simulink model "RefModel_magCalib_memoryGood"  (R2020b)
settings: Solver=FixedStepDiscrete  StartTime=0.0  StopTime=inf  FixedStep=Ts  RelTol=1e-3
model workspace (MAT data in the model file):
  Tf = 231.9
  Ts = 0.012
  xSim1.time = [0 0.012 0.024 0.036 0.048 0.06 0.072 0.084 0.096 0.108 0.12 0.132 ... (19326 elements, 1x19326)]
  xSim1.signals.values = [0.0833129882812 0.0833129882812 0.078857421875 0.0801391601562 0.0801391601562 0.07763671875 0.07470703125 0.07470703125 0.0751342773438 0.07763671875 0.07763671875 0.0755615234375 ... (57978 elements, 19326x3)]
  xSim1.signals.dimensions = 3
  xSim2.time = [0 0.012 0.024 0.036 0.048 0.06 0.072 0.084 0.096 0.108 0.12 0.132 ... (19326 elements, 1x19326)]
  xSim2.signals.values = [0.167907714844 0.167907714844 0.176208496094 0.172912597656 0.172912597656 0.17431640625 0.178894042969 0.178894042969 0.174743652344 0.173278808594 0.173278808594 0.176208496094 ... (57978 elements, 19326x3)]
  xSim2.signals.dimensions = 3
settings Model: PauseTimes=66  PacingRate=0.011000  Creator=sl  LastModifiedBy=sl
settings OptimizationCC: DefaultParameterBehavior=Inlined  EnhancedBackFolding=on  PassReuseOutputArgsAs=Individual arguments  ZeroExternalMemoryAtStartup=off  ZeroInternalMemoryAtStartup=off  MaxStackSize=64  OptimizeBlockOrder=speed  DifferentSizesBufferReuse=on  OptimizationCustomize=off  EfficientTunableParamExpr=on
settings DebuggingCC: ParameterTunabilityLossMsg=error
settings HardwareCC: ProdBitPerPointer=32  ProdBitPerSizeT=32  ProdBitPerPtrDiffT=32  ProdLargestAtomicInteger=Long  ProdLargestAtomicFloat=Double  ProdWordSize=32  ProdHWDeviceType=ARM Compatible->ARM Cortex
settings SFSimCC: MATLABDynamicMemAlloc=off
settings RTWCC: Description=Embedded Coder  SystemTargetFile=ert.tlc  GenCodeOnly=on  PackageGeneratedCodeAndArtifacts=on  TemplateMakefile=ert_default_tmf  GenerateReport=on  IncludeHyperlinkInReport=on  LaunchReport=on  GenerateTraceInfo=on  GenerateTraceReport=on  GenerateTraceReportSl=on  GenerateTraceReportSf=on  GenerateTraceReportEml=on
settings CodeAppCC: ForceParamTrailComments=on  IgnoreCustomStorageClasses=off  OperatorAnnotations=on  SimulinkDataObjDesc=on  SFDataObjDesc=on  InsertBlockDesc=on
settings ERTTargetCC: SupportVariableSizeSignals=on  ERTCustomFileTemplate=example_file_process.tlc  ERTFilePackagingFormat=Compact

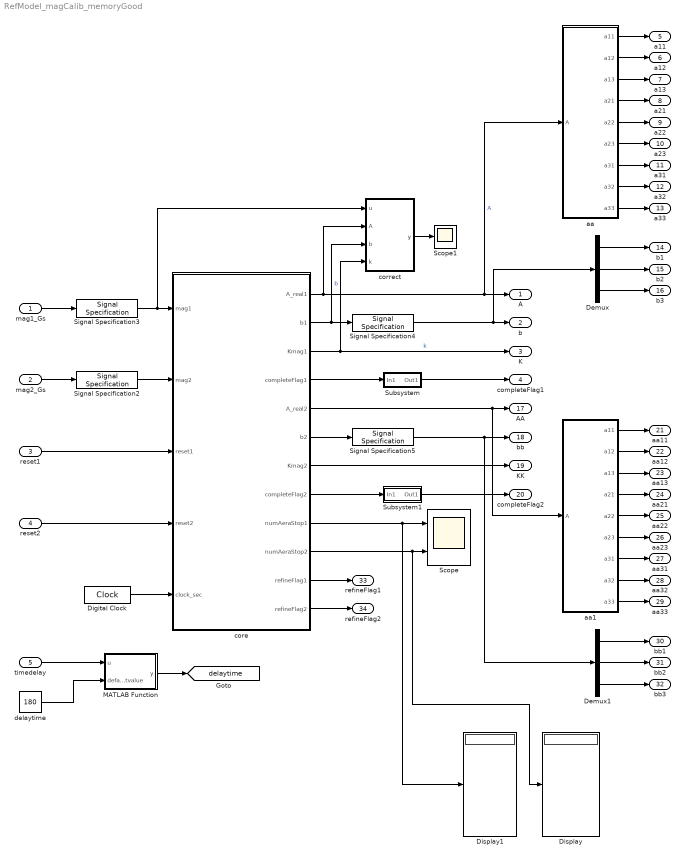
== system RefModel_magCalib_memoryGood ==
  mag1_Gs : Inport
  mag2_Gs : Inport  Port=2
  reset1 : Inport  Port=3
  reset2 : Inport  Port=4
  timedelay : Inport  Port=5
  Demux : Demux  Outputs=3
  Demux1 : Demux  Outputs=3
  Digital Clock : DigitalClock  SampleTime=-1
  Display : Display
  Display1 : Display
  MATLAB Function : MATLAB Function  TreatAsAtomicUnit=on
  Scope : Scope  NumInputPorts=2
  Scope1 : Scope
  Signal Specification{2..5} (4 alike) : SignalSpecification  OutDataTypeStr=single  Dimensions=[1,3]
  Subsystem : Subsystem
  Subsystem1 : Subsystem
  aa : MATLAB Function  TreatAsAtomicUnit=on
  aa1 : MATLAB Function  TreatAsAtomicUnit=on
  core : MATLAB Function  TreatAsAtomicUnit=on
  correct : MATLAB Function  TreatAsAtomicUnit=on
  delaytime : Constant  Value=180
  A : Outport
  b : Outport  Port=2
  K : Outport  Port=3
  completeFlag1 : Outport  Port=4
  a11 : Outport  Port=5
  a12 : Outport  Port=6
  a13 : Outport  Port=7
  a21 : Outport  Port=8
  a22 : Outport  Port=9
  a23 : Outport  Port=10
  a31 : Outport  Port=11
  a32 : Outport  Port=12
  a33 : Outport  Port=13
  b1 : Outport  Port=14
  b2 : Outport  Port=15
  b3 : Outport  Port=16
  AA : Outport  Port=17
  bb : Outport  Port=18
  KK : Outport  Port=19
  completeFlag2 : Outport  Port=20
  aa11 : Outport  Port=21
  aa12 : Outport  Port=22
  aa13 : Outport  Port=23
  aa21 : Outport  Port=24
  aa22 : Outport  Port=25
  aa23 : Outport  Port=26
  aa31 : Outport  Port=27
  aa32 : Outport  Port=28
  aa33 : Outport  Port=29
  bb1 : Outport  Port=30
  bb2 : Outport  Port=31
  bb3 : Outport  Port=32
  refineFlag1 : Outport  Port=33
  refineFlag2 : Outport  Port=34
  tag scope: delaytime=global
  wires:
  aa/2(a12) -> a12/1
  Signal Specification3/1 -> correct/1(u), core/1(mag1)
  aa/3(a13) -> a13/1
  core/1(A_real1) -> correct/2(A), aa/1(A), A/1  "A"
  aa/4(a21) -> a21/1
  core/4(completeFlag1) -> Subsystem/1(In1)
  aa/5(a22) -> a22/1
  aa/9(a33) -> a33/1
  Demux/3 -> b3/1
  Demux/1 -> b1/1
  Demux/2 -> b2/1
  aa/6(a23) -> a23/1
  aa/7(a31) -> a31/1
  aa/1(a11) -> a11/1
  core/2(b1) -> correct/3(b), Signal Specification4/1  "b"
  aa/8(a32) -> a32/1
  mag1_Gs/1 -> Signal Specification3/1
  core/3(Kmag1) -> correct/4(k), K/1  "k"
  Signal Specification2/1 -> core/2(mag2)
  mag2_Gs/1 -> Signal Specification2/1
  core/7(Kmag2) -> KK/1
  core/8(completeFlag2) -> Subsystem1/1(In1)
  aa1/3(a13) -> aa13/1
  core/6(b2) -> Signal Specification5/1
  aa1/4(a21) -> aa21/1
  aa1/9(a33) -> aa33/1
  aa1/5(a22) -> aa22/1
  aa1/8(a32) -> aa32/1
  core/5(A_real2) -> AA/1, aa1/1(A)
  aa1/7(a31) -> aa31/1
  Demux1/1 -> bb1/1
  Demux1/3 -> bb3/1
  aa1/2(a12) -> aa12/1
  Demux1/2 -> bb2/1
  aa1/1(a11) -> aa11/1
  aa1/6(a23) -> aa23/1
  reset1/1 -> core/3(reset1)
  reset2/1 -> core/4(reset2)
  Signal Specification4/1 -> Demux/1, b/1
  Signal Specification5/1 -> Demux1/1, bb/1
  core/9(numAeraStop1) -> Display1/1, Scope/1
  core/10(numAeraStop2) -> Scope/2, Display/1
  correct/1(y) -> Scope1/1
  Digital Clock/1 -> core/5(clock_sec)
  core/11(refineFlag1) -> refineFlag1/1
  core/12(refineFlag2) -> refineFlag2/1
  Subsystem/1(Out1) -> completeFlag1/1
  Subsystem1/1(Out1) -> completeFlag2/1
  timedelay/1 -> MATLAB Function/1(u)
  MATLAB Function/1(y) -> [delaytime]
  delaytime/1 -> MATLAB Function/2(defaultvalue)

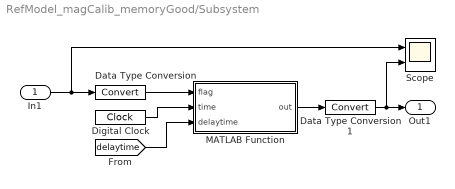
== system RefModel_magCalib_memoryGood/Subsystem ==
  In1 : Inport
  Data Type Conversion : DataTypeConversion
  Data Type Conversion1 : DataTypeConversion
  Digital Clock : DigitalClock  SampleTime=-1
  MATLAB Function : MATLAB Function  TreatAsAtomicUnit=on
  Scope : Scope  NumInputPorts=2
  Out1 : Outport
  wires:
  In1/1 -> Scope/1, Data Type Conversion/1
  MATLAB Function/1(out) -> Data Type Conversion1/1
  Digital Clock/1 -> MATLAB Function/2(time)
  Data Type Conversion/1 -> MATLAB Function/1(flag)
  Data Type Conversion1/1 -> Scope/2, Out1/1
  [delaytime] -> MATLAB Function/3(delaytime)

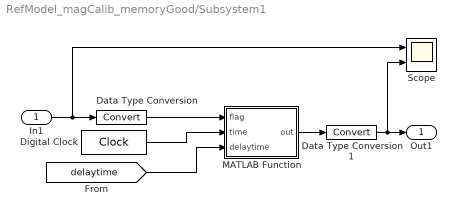
== system RefModel_magCalib_memoryGood/Subsystem1 ==
  In1 : Inport
  Data Type Conversion : DataTypeConversion
  Data Type Conversion1 : DataTypeConversion
  Digital Clock : DigitalClock  SampleTime=-1
  MATLAB Function : MATLAB Function  TreatAsAtomicUnit=on
  Scope : Scope  NumInputPorts=2
  Out1 : Outport
  wires:
  In1/1 -> Scope/1, Data Type Conversion/1
  MATLAB Function/1(out) -> Data Type Conversion1/1
  Digital Clock/1 -> MATLAB Function/2(time)
  Data Type Conversion/1 -> MATLAB Function/1(flag)
  Data Type Conversion1/1 -> Scope/2, Out1/1
  [delaytime] -> MATLAB Function/3(delaytime)

== matlab function RefModel_magCalib_memoryGood/MATLAB Function ==
  data: u input; y output; defaultvalue input
function y = fcn(u,defaultvalue)
if u == 0
    y = defaultvalue;
else
    y = u;
end

== matlab function RefModel_magCalib_memoryGood/aa1 ==
  data: A input; a11 output; a12 output; a13 output; a21 output; a22 output; a23 output; a31 output; a32 output; a33 output
function [a11,a12,a13,a21,a22,a23,a31,a32,a33] = fcn(A)
a11 = A(1,1);
a12 = A(1,2);
a13 = A(1,3);
a21 = A(2,1);
a22 = A(2,2);
a23 = A(2,3);
a31 = A(3,1);
a32 = A(3,2);
a33 = A(3,3);

== matlab function RefModel_magCalib_memoryGood/correct ==
  data: u input; y output; A input; b input; k input
function y = fcn(u, A, b, k)
u = k*(u-b)*A;
y = norm(u);

== matlab function RefModel_magCalib_memoryGood/Subsystem/MATLAB Function ==
  data: flag input; out output; time input; delaytime input
function out = fcn(flag,time, delaytime)
persistent preflag timeflag
if isempty(preflag)
    preflag = 0;
    timeflag = inf;
end
if preflag == 0 && flag ~= 0
    timeflag = time;
end
% slassddd
if (time-timeflag) > delaytime
    out = 1;
else
    out = 0;
end
preflag = flag;

== matlab function RefModel_magCalib_memoryGood/aa ==
  data: A input; a11 output; a12 output; a13 output; a21 output; a22 output; a23 output; a31 output; a32 output; a33 output
function [a11,a12,a13,a21,a22,a23,a31,a32,a33] = fcn(A)
a11 = A(1,1);
a12 = A(1,2);
a13 = A(1,3);
a21 = A(2,1);
a22 = A(2,2);
a23 = A(2,3);
a31 = A(3,1);
a32 = A(3,2);
a33 = A(3,3);

== matlab function RefModel_magCalib_memoryGood/core ==
  data: A_real1 output; b1 output; Kmag1 output; mag1 input; completeFlag1 output; A_real2 output; b2 output; Kmag2 output; completeFlag2 output; numAeraStop1 output; numAeraStop2 output; mag2 input; reset1 input; reset2 input; clock_sec input; refineFlag1 output; refineFlag2 output
function [A_real1,b1,Kmag1,completeFlag1,...
    A_real2,b2,Kmag2,completeFlag2,numAeraStop1,numAeraStop2,refineFlag1,refineFlag2] = fcn(mag1,mag2,reset1,reset2,clock_sec)
persistent refine1 refine2 pb1 pb2
if isempty(refine1)
    refine1 = false;
    refine2 = false;
    pb1 = single(zeros(1,3));
    pb2 = single(zeros(1,3));
end
enableRefine = true;
if refine1
    mag1 = mag1 - pb1;
end
if refine2
    mag2 = mag2 - pb2;
end
[A_real1,b1,Kmag1,completeFlag1,numAeraStop1] = calMag1(mag1,reset1,pb1);
[A_real2,b2,Kmag2,completeFlag2,numAeraStop2] = calMag2(mag2,reset2,pb2);
n1 = sum(numAeraStop1~=0);
n2 = sum(numAeraStop2~=0);
if enableRefine
    if n1 == 8 && ~completeFlag2 && refine2
    %     磁力计2所处磁场可能较差
        fprintf('%.2f sec: mag2 is going to refined --------------------------------------------------------\n',clock_sec);
        refine2 = true;
        pb2 = b2;
    end
    if n2 == 8 && ~completeFlag1 && ~refine1
    %     磁力计1所处磁场可能较差
        fprintf('%.2f sec: mag1 is going to refined --------------------------------------------------------\n',clock_sec);
        refine1 = true;
        pb1 = b1;
    end
end

if refine1
    b1 = b1 + pb1;
end
if refine2
    b2 = b2 + pb2;
end
refineFlag1 = refine1;
refineFlag2 = refine2;
end

% function flag = detectNotUpdate(mag,magpre)
% flag = false;
% if isequal(mag,magpre)
%     flag = true;
% end
% end
%% 子函数
% mag2
function [A_real,b,Kmag,completeFlag,numAeraStop_out] = calMag2(mag,reset,db)
persistent m2_step m2_A_p m2_b_p m2_Kmag_p m2_mag_pre m2_completeFlag_p m2_preDb
persistent m2_aera1 m2_aera2 m2_aera3 m2_aera4 m2_aera5 m2_aera6 m2_aera7 m2_aera8
persistent m2_numAeraStop m2_numAeraStopPre
magNum = int16(2);
maxNumInAera = 5;
emptyVecFlag = single(9999*[1 1 1]); % 占位向量，视为无效数据
nArea = 8;
maxNum = single(nArea*maxNumInAera);  % 最大数据维数
if isempty(m2_step) || reset
    m2_step = single(0);
    m2_A_p = single(eye(3));
    m2_b_p = single(zeros(1,3));
    m2_Kmag_p = single(1);
    m2_mag_pre = single(zeros(1,3));
    m2_completeFlag_p = single(0);
    
    [m2_aera1,m2_aera2,m2_aera3,m2_aera4,m2_aera5,m2_aera6,m2_aera7,m2_aera8] = resetAreaData(emptyVecFlag,maxNumInAera);
    
    m2_numAeraStop = zeros(1,nArea);
    m2_numAeraStopPre = zeros(1,nArea);
    m2_preDb = db;
end
if sum(abs(m2_preDb)) == 0 && sum(abs(db)) ~= 0
    [m2_aera1,m2_aera2,m2_aera3,m2_aera4,m2_aera5,m2_aera6,m2_aera7,m2_aera8] = correctAreaDataBuffer(db,m2_preDb,maxNumInAera,emptyVecFlag,...
        m2_aera1,m2_aera2,m2_aera3,m2_aera4,m2_aera5,m2_aera6,m2_aera7,m2_aera8);
end
m2_preDb = db;

numAeraStop_out = m2_numAeraStop;
m2_step = m2_step + 1;
% 预置值
A_real = m2_A_p;
b = m2_b_p;
Kmag = m2_Kmag_p;
completeFlag = m2_completeFlag_p;
% 收集数据
numStop = maxNum;
dmag = norm(m2_mag_pre-mag);
%% 更新采集点
limit = max(min(0.5,norm(mag)),0.2);
updateEnable = dmag>limit;
if updateEnable %rem(step,50) == 0
    % 保存点
    [m2_mag_pre,m2_numAeraStop,m2_aera1,m2_aera2,m2_aera3,m2_aera4,m2_aera5,m2_aera6,m2_aera7,m2_aera8] = ...
        allocData(mag,emptyVecFlag,maxNumInAera,nArea,m2_numAeraStop,m2_aera1,m2_aera2,m2_aera3,m2_aera4,m2_aera5,m2_aera6,m2_aera7,m2_aera8);
    % 判断采样点是否积累到一定数量
    allDataNum = sum(m2_numAeraStop);
    aeraValid = zeros(1,nArea);
    for i = 1:nArea
        aeraValid(i) = m2_numAeraStop(i)>0;
    end
    if ~isequal(m2_numAeraStopPre, m2_numAeraStop)
                fprintf('Mag%d [%d %d %d %d %d %d %d %d]\n ',int16(magNum),...
                    int16(m2_numAeraStop(1)),int16(m2_numAeraStop(2)),int16(m2_numAeraStop(3)),int16(m2_numAeraStop(4)),...
                    int16(m2_numAeraStop(5)),int16(m2_numAeraStop(6)),int16(m2_numAeraStop(7)),int16(m2_numAeraStop(8)));     
    end
    m2_numAeraStopPre = m2_numAeraStop;    
    if allDataNum < maxNum*2/3 || sum(aeraValid) < 6
%         return;
    end
    if false
        printAreaData(2,maxNumInAera,m2_aera1,m2_aera2,m2_aera3,m2_aera4,m2_aera5,m2_aera6,m2_aera7,m2_aera8);
    end    
else
    return;
end

% ---------------------
%%
% 进行椭圆矫正参数计算
allData = getAllData(emptyVecFlag,maxNumInAera,nArea,...
    m2_aera1,m2_aera2,m2_aera3,m2_aera4,m2_aera5,m2_aera6,m2_aera7,m2_aera8);
% [A,bCol,magB] = bestfit(dataRecord(1:numStop,1),dataRecord(1:numStop,2),dataRecord(1:numStop,3));
allDataNum = sum(m2_numAeraStop);
[A,bCol,magB] = bestfit(allData(1:allDataNum,1),allData(1:allDataNum,2),allData(1:allDataNum,3));
bCol = real(bCol);
A_real = real(A);
Kmag = 0.54/real(magB);
b = bCol(:).'; % make a row vector
% 矫正公式：x_correct =（x-b）*A;
%     x_correct = bsxfun(@minus,mag,b)*A_real;

m2_A_p = A;
m2_b_p = b;
m2_Kmag_p = Kmag;

if ~isdiag(A) && allDataNum > maxNum*2/3 || sum(aeraValid) >= 6
    m2_completeFlag_p = single(1);
end
if  ~isdiag(A) && all(aeraValid>1) && allDataNum > maxNum*4/5
    m2_completeFlag_p = single(2);    
end
completeFlag = m2_completeFlag_p;
%     scatter3(dataRecord(1:numStop,1),dataRecord(1:numStop,2),dataRecord(1:numStop,3),'r');axis equal;
end
% mag1
function [A_real,b,Kmag,completeFlag,numAeraStop_out] = calMag1(mag,reset,db)
persistent m1_step m1_A_p m1_b_p m1_Kmag_p m1_mag_pre m1_completeFlag_p m1_preDb
persistent m1_aera1 m1_aera2 m1_aera3 m1_aera4 m1_aera5 m1_aera6 m1_aera7 m1_aera8
persistent m1_numAeraStop m1_numAeraStopPre
magNum = int16(1);
maxNumInAera = 5;
emptyVecFlag = single(9999*[1 1 1]); % 占位向量，视为无效数据
nArea = 8;
maxNum = single(nArea*maxNumInAera);  % 最大数据维数
if isempty(m1_step) || reset
    m1_step = single(0);
    m1_A_p = single(eye(3));
    m1_b_p = single(zeros(1,3));
    m1_Kmag_p = single(1);
    m1_mag_pre = single(zeros(1,3));
    m1_completeFlag_p = single(0);
    
    [m1_aera1,m1_aera2,m1_aera3,m1_aera4,m1_aera5,m1_aera6,m1_aera7,m1_aera8] = resetAreaData(emptyVecFlag,maxNumInAera);
    
    m1_numAeraStop = zeros(1,nArea);
    m1_numAeraStopPre = zeros(1,nArea);
    m1_preDb = db;
end
if sum(abs(m1_preDb)) == 0 && sum(abs(db)) ~= 0
    [m1_aera1,m1_aera2,m1_aera3,m1_aera4,m1_aera5,m1_aera6,m1_aera7,m1_aera8] = correctAreaDataBuffer(db,m1_preDb,maxNumInAera,emptyVecFlag,...
        m1_aera1,m1_aera2,m1_aera3,m1_aera4,m1_aera5,m1_aera6,m1_aera7,m1_aera8);
    % 将 areaN 中的数据提取至 allData
    allData = getAllData(emptyVecFlag,maxNumInAera,nArea,...
        m1_aera1,m1_aera2,m1_aera3,m1_aera4,m1_aera5,m1_aera6,m1_aera7,m1_aera8);
    % 清空 areaN 
    [m1_aera1,m1_aera2,m1_aera3,m1_aera4,m1_aera5,m1_aera6,m1_aera7,m1_aera8] = resetAreaData(emptyVecFlag,maxNumInAera);
    % 重新将矫正后的数据赋值给 areaN
    for i = 1:maxNumInAera*nArea
        tempMag = allData(i,:);
        if tempMag(1) ~= emptyVecFlag(1)
            % 有效数据
            [m1_mag_pre,m1_numAeraStop,m1_aera1,m1_aera2,m1_aera3,m1_aera4,m1_aera5,m1_aera6,m1_aera7,m1_aera8] = ...
                allocData(tempMag,emptyVecFlag,maxNumInAera,nArea,m1_numAeraStop,m1_aera1,m1_aera2,m1_aera3,m1_aera4,m1_aera5,m1_aera6,m1_aera7,m1_aera8);
        end
    end
end
m1_preDb = db;
numAeraStop_out = m1_numAeraStop;
m1_step = m1_step + 1;
% 预置值
A_real = m1_A_p;
b = m1_b_p;
Kmag = m1_Kmag_p;
completeFlag = m1_completeFlag_p;
% 收集数据
numStop = maxNum;
dmag = norm(m1_mag_pre-mag);
%% 更新采集点
limit = max(min(0.5,norm(mag)),0.2);
updateEnable = dmag>limit;
if updateEnable %rem(step,50) == 0
    % 保存点
    [m1_mag_pre,m1_numAeraStop,m1_aera1,m1_aera2,m1_aera3,m1_aera4,m1_aera5,m1_aera6,m1_aera7,m1_aera8] = ...
        allocData(mag,emptyVecFlag,maxNumInAera,nArea,m1_numAeraStop,m1_aera1,m1_aera2,m1_aera3,m1_aera4,m1_aera5,m1_aera6,m1_aera7,m1_aera8);
    % 判断采样点是否积累到一定数量
    allDataNum = sum(m1_numAeraStop);
    aeraValid = zeros(1,nArea);
    for i = 1:nArea
        aeraValid(i) = m1_numAeraStop(i)>0;
    end
    if ~isequal(m1_numAeraStopPre, m1_numAeraStop)
                fprintf('Mag%d [%d %d %d %d %d %d %d %d]\n ',int16(magNum),...
                    int16(m1_numAeraStop(1)),int16(m1_numAeraStop(2)),int16(m1_numAeraStop(3)),int16(m1_numAeraStop(4)),...
                    int16(m1_numAeraStop(5)),int16(m1_numAeraStop(6)),int16(m1_numAeraStop(7)),int16(m1_numAeraStop(8)));     
    end
    m1_numAeraStopPre = m1_numAeraStop;    
    if allDataNum < maxNum*2/3 || sum(aeraValid) < 6
%         return;
    end
    if false
        printAreaData(1,maxNumInAera,m1_aera1,m1_aera2,m1_aera3,m1_aera4,m1_aera5,m1_aera6,m1_aera7,m1_aera8);
    end    
else
    return;
end

% ---------------------
%%
% 进行椭圆矫正参数计算
allData = getAllData(emptyVecFlag,maxNumInAera,nArea,...
    m1_aera1,m1_aera2,m1_aera3,m1_aera4,m1_aera5,m1_aera6,m1_aera7,m1_aera8);
% [A,bCol,magB] = bestfit(dataRecord(1:numStop,1),dataRecord(1:numStop,2),dataRecord(1:numStop,3));
allDataNum = sum(m1_numAeraStop);
[A,bCol,magB] = bestfit(allData(1:allDataNum,1),allData(1:allDataNum,2),allData(1:allDataNum,3));
bCol = real(bCol);
A_real = real(A);
Kmag = 0.54/real(magB);
b = bCol(:).'; % make a row vector
% 矫正公式：x_correct =（x-b）*A;
%     x_correct = bsxfun(@minus,mag,b)*A_real;

m1_A_p = A;
m1_b_p = b;
m1_Kmag_p = Kmag;

if ~isdiag(A) && allDataNum > maxNum*2/3 || sum(aeraValid) >= 6
    m1_completeFlag_p = single(1);
end
if  ~isdiag(A) && all(aeraValid>1) && allDataNum > maxNum*4/5
    m1_completeFlag_p = single(2);    
end
completeFlag = m1_completeFlag_p;
%     scatter3(dataRecord(1:numStop,1),dataRecord(1:numStop,2),dataRecord(1:numStop,3),'r');axis equal;
end

function [A,b,magB,er] = bestfit(x,y,z)
% 在三种拟合结果中选择最佳值 （4, 7 or 10 parameter），若需降低计算量，
% 可选择其中一种计算方法

[A,b,magB, er] = correctEllipsoid4(x,y,z);

%     [A7,b7,magB7, er7, ispd7] = correctEllipsoid7(x,y,z);
%     if ispd7 && isreal(sum(imag(A7(:)))) && (er7 < er)
%         A = real(A7);
%         b = real(b7);
%         magB = magB7;
%         er = er7;
%     end

[A10,b10,magB10, er10, ispd10] = correctEllipsoid10(x,y,z);
if ispd10 && isreal(sum(imag(A10(:)))) && (er10 < er)
    A = real(A10);
    b = real(b10);
    magB = magB10;
    er = er10;
end
end

function [Winv, V,B, er, ispd] = correctEllipsoid4(x,y,z)
% R is the identity

bv = x.*x + y.*y + z.*z;

A3 = [x,y,z];
A = [A3 ones(numel(x),1, 'like', x)];

soln = A\bv;
Winv = eye(3, 'like', x);
V = 0.5*soln(1:3);
B = sqrt(soln(4) + sum(V.*V));

if nargout > 3
    res = A*soln - bv;
    er = (1/(2*B*B) * sqrt( res.'*res / numel(x)));
    ispd = 1;
else
    er = -ones(1, 'like',x);
    ispd = -1;
end
er = real(er);
end

function [Winv, V,B,er, ispd] = correctEllipsoid10(x,y,z)

d = [...
    x.*x, ...
    2*x.*y, ...
    2*x.*z, ...
    y.*y, ...
    2*y.*z, ...
    z.*z, ...
    x, ...
    y, ...
    z, ...
    ones(size(x))];

dtd = d.' * d;

[evc, evlmtx] = eig(dtd);

eigvals = diag(real(evlmtx));
[~, idx] = min(real(eigvals));

beta = real(evc(:,idx)); %solution has smallest eigenvalue

A = beta([1 2 3; 2 4 5; 3 5 6]); %make symmetric
dA = real(det(A));

if dA < 0
    A = -A;
    beta = -beta;
    dA = -dA; %Compensate for -A.
end

V = -0.5*(A\beta(7:9)); %hard iron offset

B = sqrt(abs(sum([...
    A(1,1)*V(1)*V(1), ...
    2*A(2,1)*V(2)*V(1), ...
    2*A(3,1)*V(3)*V(1), ...
    A(2,2)*V(2)*V(2), ...
    2*A(3,2)*V(2)*V(3), ...
    A(3,3)*V(3)*V(3), ...
    -beta(end)] ...
    )));

% We correct Winv and B by det(A) because we don't know which has the
% gain. By convention, normalize A.

det3root = nthroot(dA,3);
det6root = sqrt(det3root);
Winv = sqrtm(A./det3root);
B = B./det6root;

if nargout > 3
    res = residual(Winv,V,B, [x,y,z]);
    er = (1/(2*B*B))*sqrt(res.'*res/numel(x));
    [~,p] = chol(A);
    ispd = (p == 0);
else
    er = -ones(1, 'like',x);
    ispd = -1;
end
er = real(er);

end

function [Winv, V,B,er, ispd] = correctEllipsoid7(x,y,z)

d = [...
    x.*x, ...
    y.*y, ...
    z.*z, ...
    x, ...
    y, ...
    z, ...
    ones(size(x))];


dtd = d.' * d;

[evc, evlmtx] = eig(dtd);

eigvals = diag(evlmtx);
[~, idx] = min(eigvals);

beta = evc(:,idx); %solution has smallest eigenvalue
A = diag(beta(1:3));
dA = real(det(A));

if dA < 0
    A = -A;
    beta = -beta;
    dA = -dA; %Compensate for -A.
end
V = -0.5*(beta(4:6)./beta(1:3)); %hard iron offset

B = sqrt(abs(sum([...
    A(1,1)*V(1)*V(1), ...
    A(2,2)*V(2)*V(2), ...
    A(3,3)*V(3)*V(3), ...
    -beta(end)] ...
    )));


% We correct Winv and B by det(A) because we don't know which has the
% gain. By convention, normalize A.

det3root = nthroot(dA,3);
det6root = sqrt(det3root);
Winv = sqrtm(A./det3root);
B = B./det6root;

if nargout > 3
    res = residual(Winv,V,B, [x,y,z]);
    er = (1/(2*B*B))*sqrt(res.'*res/numel(x));
    [~,p] = chol(A);
    ispd = (p == 0);
else
    er = -ones(1, 'like',x);
    ispd = -1;
end
er = real(er);
end

function r = residual(Winv, V, B, data)
% Residual error after correction

spherept = (Winv * bsxfun(@minus,data.',V)).'; % a point on the unit sphere
radsq = sum(spherept.^2,2);

r = radsq - B.^2;
end

function allData = getAllData(emptyVecFlag,maxNumInAera,nArea,...
    m2_aera1,m2_aera2,m2_aera3,m2_aera4,m2_aera5,m2_aera6,m2_aera7,m2_aera8)
allData = single(emptyVecFlag(1)*ones(maxNumInAera*nArea,3));
idx = 1;
idxAllData = 1;
for i = 1:maxNumInAera*nArea
    switch ceil(i/maxNumInAera)
        case 1
            if ~isequal(m2_aera1(idx,:),emptyVecFlag)
                allData(idxAllData,:) = m2_aera1(idx,:);
                idxAllData = idxAllData+1;
            end
        case 2
            if ~isequal(m2_aera2(idx,:),emptyVecFlag)
                allData(idxAllData,:) = m2_aera2(idx,:);
                idxAllData = idxAllData+1;
            end
        case 3
            if ~isequal(m2_aera3(idx,:),emptyVecFlag)
                allData(idxAllData,:) = m2_aera3(idx,:);
                idxAllData = idxAllData+1;
            end
        case 4
            if ~isequal(m2_aera4(idx,:),emptyVecFlag)
                allData(idxAllData,:) = m2_aera4(idx,:);
                idxAllData = idxAllData+1;
            end
        case 5
            if ~isequal(m2_aera5(idx,:),emptyVecFlag)
                allData(idxAllData,:) = m2_aera5(idx,:);
                idxAllData = idxAllData+1;
            end
        case 6
            if ~isequal(m2_aera6(idx,:),emptyVecFlag)
                allData(idxAllData,:) = m2_aera6(idx,:);
                idxAllData = idxAllData+1;
            end
        case 7
            if ~isequal(m2_aera7(idx,:),emptyVecFlag)
                allData(idxAllData,:) = m2_aera7(idx,:);
                idxAllData = idxAllData+1;
            end
        case 8
            if ~isequal(m2_aera8(idx,:),emptyVecFlag)
                allData(idxAllData,:) = m2_aera8(idx,:);
                idxAllData = idxAllData+1;
            end
        otherwise
            error('error');
    end
    idx = idx + 1;
    if rem(i,maxNumInAera) == 0
        idx = 1;
    end
end
end
%
function [m1_mag_pre,m1_numAeraStop,m1_aera1,m1_aera2,m1_aera3,m1_aera4,m1_aera5,m1_aera6,m1_aera7,m1_aera8] = ...
    allocData(mag,emptyVecFlag,maxNumInAera,nArea,m1_numAeraStop,m1_aera1,m1_aera2,m1_aera3,m1_aera4,m1_aera5,m1_aera6,m1_aera7,m1_aera8)
m1_mag_pre = mag;
magx = mag(1);
magy = mag(2);
magz = mag(3);
flag_1 = magx > 0 && magy > 0 && magz >0;
flag_2 = magx > 0 && magy > 0 && magz <0;
flag_3 = magx > 0 && magy < 0 && magz >0;
flag_4 = magx > 0 && magy < 0 && magz <0;
flag_5 = magx < 0 && magy > 0 && magz >0;
flag_6 = magx < 0 && magy > 0 && magz <0;
flag_7 = magx < 0 && magy < 0 && magz >0;
flag_8 = magx < 0 && magy < 0 && magz <0;
% 分区存储
if flag_1
    m1_aera1(2:maxNumInAera,:) = m1_aera1(1:maxNumInAera-1,:);
    m1_aera1(1,:) = mag;
    for i = 1:maxNumInAera
        if isequal(m1_aera1(i,:),emptyVecFlag)
            break;
        else
            m1_numAeraStop(1) = i;
        end
    end
elseif flag_2
    m1_aera2(2:maxNumInAera,:) = m1_aera2(1:maxNumInAera-1,:);
    m1_aera2(1,:) = mag;
    for i = 1:maxNumInAera
        if isequal(m1_aera2(i,:),emptyVecFlag)
            break;
        else
            m1_numAeraStop(2) = i;
        end
    end
elseif flag_3
    m1_aera3(2:maxNumInAera,:) = m1_aera3(1:maxNumInAera-1,:);
    m1_aera3(1,:) = mag;
    for i = 1:maxNumInAera
        if isequal(m1_aera3(i,:),emptyVecFlag)
            break;
        else
            m1_numAeraStop(3) = i;
        end
    end
elseif flag_4
    m1_aera4(2:maxNumInAera,:) = m1_aera4(1:maxNumInAera-1,:);
    m1_aera4(1,:) = mag;
    for i = 1:maxNumInAera
        if isequal(m1_aera4(i,:),emptyVecFlag)
            break;
        else
            m1_numAeraStop(4) = i;
        end
    end
elseif flag_5
    m1_aera5(2:maxNumInAera,:) = m1_aera5(1:maxNumInAera-1,:);
    m1_aera5(1,:) = mag;
    for i = 1:maxNumInAera
        if isequal(m1_aera5(i,:),emptyVecFlag)
            break;
        else
            m1_numAeraStop(5) = i;
        end
    end
elseif flag_6
    m1_aera6(2:maxNumInAera,:) = m1_aera6(1:maxNumInAera-1,:);
    m1_aera6(1,:) = mag;
    for i = 1:maxNumInAera
        if isequal(m1_aera6(i,:),emptyVecFlag)
            break;
        else
            m1_numAeraStop(6) = i;
        end
    end
elseif flag_7
    m1_aera7(2:maxNumInAera,:) = m1_aera7(1:maxNumInAera-1,:);
    m1_aera7(1,:) = mag;
    for i = 1:maxNumInAera
        if isequal(m1_aera7(i,:),emptyVecFlag)
            break;
        else
            m1_numAeraStop(7) = i;
        end
    end
else
    m1_aera8(2:maxNumInAera,:) = m1_aera8(1:maxNumInAera-1,:);
    m1_aera8(1,:) = mag;
    for i = 1:maxNumInAera
        if isequal(m1_aera8(i,:),emptyVecFlag)
            break;
        else
            m1_numAeraStop(8) = i;
        end
    end
end
end
%
function [m2_aera1,m2_aera2,m2_aera3,m2_aera4,m2_aera5,m2_aera6,m2_aera7,m2_aera8] = correctAreaDataBuffer(db,m2_preDb,maxNumInAera,emptyVecFlag,...
    m2_aera1,m2_aera2,m2_aera3,m2_aera4,m2_aera5,m2_aera6,m2_aera7,m2_aera8)
    % 在db变为非零时，aera数据执行一次操作
    for i = 1:maxNumInAera
        if m2_aera1(i,1) ~= emptyVecFlag(1)
            temp = m2_aera1(i,:) - db;
            m2_aera1(i,:) = temp;
        end
        
        if m2_aera2(i,1) ~= emptyVecFlag(1)
            temp = m2_aera2(i,:) - db;
            m2_aera2(i,:) = temp;
        end
        if m2_aera3(i,1) ~= emptyVecFlag(1)
            temp = m2_aera3(i,:) - db;
            m2_aera3(i,:) = temp;
        end
        if m2_aera4(i,1) ~= emptyVecFlag(1)
            temp = m2_aera4(i,:) - db;
            m2_aera4(i,:) = temp;
        end
        if m2_aera5(i,1) ~= emptyVecFlag(1)
            temp = m2_aera5(i,:) - db;
            m2_aera5(i,:) = temp;
        end
        if m2_aera6(i,1) ~= emptyVecFlag(1)
            temp = m2_aera6(i,:) - db;
            m2_aera6(i,:) = temp;
        end
        if m2_aera7(i,1) ~= emptyVecFlag(1)
            temp = m2_aera7(i,:) - db;
            m2_aera7(i,:) = temp;
        end
        if m2_aera8(i,1) ~= emptyVecFlag(1)
            temp = m2_aera8(i,:) - db;
            m2_aera8(i,:) = temp;
        end
        
    end
end
%
function printAreaData(idxMag,maxNumInAera,m2_aera1,m2_aera2,m2_aera3,m2_aera4,m2_aera5,m2_aera6,m2_aera7,m2_aera8)
fprintf('mag%d\n',int8(idxMag));
fprintf('\t area1:\n');
for i = 1:maxNumInAera    
    fprintf('\t\t %.2f\t%.2f\t%.2f\t\n',m2_aera1(i,1),m2_aera1(i,2),m2_aera1(i,3));
end
fprintf('\t area2:\n');
for i = 1:maxNumInAera
    fprintf('\t\t %.2f\t%.2f\t%.2f\t\n',m2_aera2(i,1),m2_aera2(i,2),m2_aera2(i,3));
end
fprintf('\t area3:\n');
for i = 1:maxNumInAera    
    fprintf('\t\t %.2f\t%.2f\t%.2f\t\n',m2_aera3(i,1),m2_aera3(i,2),m2_aera3(i,3));
end
fprintf('\t area4:\n');
for i = 1:maxNumInAera
    fprintf('\t\t %.2f\t%.2f\t%.2f\t\n',m2_aera4(i,1),m2_aera4(i,2),m2_aera4(i,3));
end
fprintf('\t area5:\n');
for i = 1:maxNumInAera    
    fprintf('\t\t %.2f\t%.2f\t%.2f\t\n',m2_aera5(i,1),m2_aera5(i,2),m2_aera5(i,3));
end
fprintf('\t area6:\n');
for i = 1:maxNumInAera    
    fprintf('\t\t %.2f\t%.2f\t%.2f\t\n',m2_aera6(i,1),m2_aera6(i,2),m2_aera6(i,3));
end
fprintf('\t area7:\n');
for i = 1:maxNumInAera    
    fprintf('\t\t %.2f\t%.2f\t%.2f\t\n',m2_aera7(i,1),m2_aera7(i,2),m2_aera7(i,3));
end
fprintf('\t area8:\n');
for i = 1:maxNumInAera    
    fprintf('\t\t %.2f\t%.2f\t%.2f\t\n',m2_aera8(i,1),m2_aera8(i,2),m2_aera8(i,3));
end
end
%
function [m2_aera1,m2_aera2,m2_aera3,m2_aera4,m2_aera5,m2_aera6,m2_aera7,m2_aera8] = resetAreaData(emptyVecFlag,maxNumInAera)
    m2_aera1 = single(emptyVecFlag(1)*ones(maxNumInAera,3));
    m2_aera2 = single(emptyVecFlag(1)*ones(maxNumInAera,3));
    m2_aera3 = single(emptyVecFlag(1)*ones(maxNumInAera,3));
    m2_aera4 = single(emptyVecFlag(1)*ones(maxNumInAera,3));
    m2_aera5 = single(emptyVecFlag(1)*ones(maxNumInAera,3));
    m2_aera6 = single(emptyVecFlag(1)*ones(maxNumInAera,3));
    m2_aera7 = single(emptyVecFlag(1)*ones(maxNumInAera,3));
    m2_aera8 = single(emptyVecFlag(1)*ones(maxNumInAera,3));
end

== matlab function RefModel_magCalib_memoryGood/Subsystem1/MATLAB Function ==
  data: flag input; out output; time input; delaytime input
function out = fcn(flag,time, delaytime)
persistent preflag timeflag
if isempty(preflag)
    preflag = 0;
    timeflag = inf;
end
if preflag == 0 && flag ~= 0
    timeflag = time;
end
% slassddd
if (time-timeflag) > delaytime
    out = 1;
else
    out = 0;
end
preflag = flag;
